simulink model "manipulacion_1_enlace_complemento"  (R2022b)
settings: Solver=VariableStepAuto  StartTime=0.0  StopTime=10  RelTol=1e-3
settings Model: Creator=alex  LastModifiedBy=alex

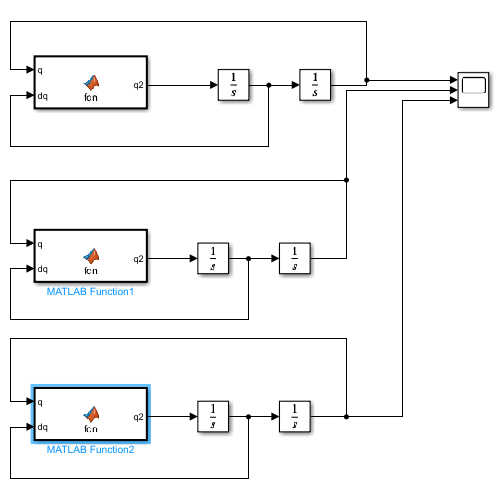
[thumbnail: Simulink's stored preview of the top-level diagram]
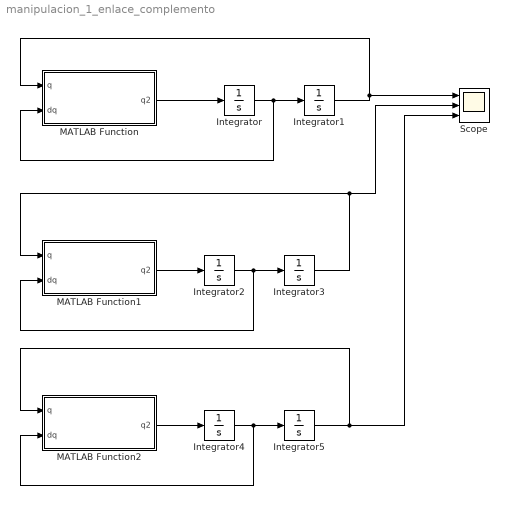
== system manipulacion_1_enlace_complemento ==
  Integrator : Integrator
  Integrator1 : Integrator  InitialCondition=2*pi
  Integrator2 : Integrator
  Integrator3 : Integrator  InitialCondition=2*pi
  Integrator4 : Integrator
  Integrator5 : Integrator  InitialCondition=2*pi
  MATLAB Function : MATLAB Function  TreatAsAtomicUnit=on
  MATLAB Function1 : MATLAB Function  TreatAsAtomicUnit=on
  MATLAB Function2 : MATLAB Function  TreatAsAtomicUnit=on
  Scope : Scope  NumInputPorts=3
  wires:
  Integrator1/1 -> Scope/1, MATLAB Function/1(q)
  Integrator/1 -> MATLAB Function/2(dq), Integrator1/1
  MATLAB Function/1(q2) -> Integrator/1
  Integrator2/1 -> MATLAB Function1/2(dq), Integrator3/1
  MATLAB Function1/1(q2) -> Integrator2/1
  Integrator3/1 -> Scope/2, MATLAB Function1/1(q)
  Integrator4/1 -> MATLAB Function2/2(dq), Integrator5/1
  MATLAB Function2/1(q2) -> Integrator4/1
  Integrator5/1 -> Scope/3, MATLAB Function2/1(q)

== matlab function manipulacion_1_enlace_complemento/MATLAB Function ==
  data: q input; q2 output; dq input
function q2 = fcn(q,dq)


k=0.5;
m = 0.75;
l=0.36
g=9.8
t = 0.1

a= l/2
j=(4/3)*(m*a*a)


q2= (-(m*g*a*cos(q))+t-(k*dq))/j

== matlab function manipulacion_1_enlace_complemento/MATLAB Function2 ==
  data: q input; q2 output; dq input
function q2 = fcn(q,dq)


k=0.5;
m = 0.75;
l=0.36
g=9.8
t = 0.1

a= l/2
j=(4/3)*(m*a*a)


q2= (-(m*g*a*(q))+t-(k*dq))/j

== matlab function manipulacion_1_enlace_complemento/MATLAB Function1 ==
  data: q input; q2 output; dq input
function q2 = fcn(q,dq)


k=0.5;
m = 0.75;
l=0.36
g=9.8
t = 0.1

a= l/2
j=(4/3)*(m*a*a)


q2= (-(m*g*a*sin(q))+t-(k*dq))/j
